simulink model "VINS"  (R2018a)
settings: Solver=FixedStepDiscrete  StartTime=0.0  StopTime=inf  FixedStep=1/Fs  RelTol=1e-3  EnableMultiTasking=on
PreLoadFcn:
  | modelDef = getModelDef(calibrateSFMA);
  | 
  | %imuPar = getImuPar('lmvpUncalibrated');
  | 
  | timeMatchThreshold = 1000;
undefined symbols (not defined in the file or in its folder): beep, dejitter_on, Fs, homogeneous3x4Transform_k_kmin1, imuLocationMm, imuPar, numStates, simData, tstamp_k_us, tstamp_kmin1_us
libraries: simulink x69, dspmtrx3 x35, dspindex x9, vrlib x7, dspstat3 x7, dspinverses x6, dspsigops x5, dspmathops x2, rtwdemowidgets x1, dspfactors x1, simulink_extras x1
(part 4 of 6)

== system VINS/measUpdate/plotVidLatency/DT convert ==
  In1 : Inport
  Data Store Read : DataStoreRead  DataStoreName=DataTypeRef
  Data Type Conversion Inherited : simulink/Signal Attributes/Data Type Conversion Inherited  ConvertRealWorld=Real World Value  DoSatur=off
      settings: SourceProductName=Simulink  SourceProductBaseCode=SL
  Out1 : Outport
  wires:
  Data Type Conversion Inherited/1 -> Out1/1
  Data Store Read/1 -> Data Type Conversion Inherited/1
  In1/1 -> Data Type Conversion Inherited/2

== system VINS/measUpdate/plotVidLatency/DT convert1 ==
  In1 : Inport
  Data Store Read : DataStoreRead  DataStoreName=DataTypeRef
  Data Type Conversion Inherited : simulink/Signal Attributes/Data Type Conversion Inherited  ConvertRealWorld=Real World Value  DoSatur=off
      settings: SourceProductName=Simulink  SourceProductBaseCode=SL
  Out1 : Outport
  wires:
  In1/1 -> Data Type Conversion Inherited/2
  Data Store Read/1 -> Data Type Conversion Inherited/1
  Data Type Conversion Inherited/1 -> Out1/1

== system VINS/measUpdate/plotVidLatency/DT convert2 ==
  In1 : Inport
  Data Store Read : DataStoreRead  DataStoreName=DataTypeRef
  Data Type Conversion Inherited : simulink/Signal Attributes/Data Type Conversion Inherited  ConvertRealWorld=Real World Value  DoSatur=off
      settings: SourceProductName=Simulink  SourceProductBaseCode=SL
  Out1 : Outport
  wires:
  In1/1 -> Data Type Conversion Inherited/2
  Data Store Read/1 -> Data Type Conversion Inherited/1
  Data Type Conversion Inherited/1 -> Out1/1

== system VINS/measUpdate/plotVidLatency/set 0x08 bit ==
  Enable : EnablePort
  Assertion : Assertion  AssertionFailFcn=disp('Unacceptable video delay >3 frames'); beep;  StopWhenAssertionFail=off
  Bit Set : simulink/Logic and Bit Operations/Bit Set  iBit=3
      settings: SourceProductName=Simulink  SourceProductBaseCode=SL
  Constant : Constant  Value=false
  Data Store Read : DataStoreRead  DataStoreName=errorBitfield
  Data Store Write : DataStoreWrite  DataStoreName=errorBitfield
  wires:
  Data Store Read/1 -> Bit Set/1
  Bit Set/1 -> Data Store Write/1
  Constant/1 -> Assertion/1

== system VINS/measUpdate/plotVidLatency/set 0x10 bit ==
  Enable : EnablePort
  Assertion : Assertion  AssertionFailFcn=disp('Unacceptable video delay >3.9 frames'); beep;  StopWhenAssertionFail=off
  Bit Set : simulink/Logic and Bit Operations/Bit Set  iBit=4
      settings: SourceProductName=Simulink  SourceProductBaseCode=SL
  Constant : Constant  Value=false
  Data Store Read : DataStoreRead  DataStoreName=errorBitfield
  Data Store Write : DataStoreWrite  DataStoreName=errorBitfield
  wires:
  Constant/1 -> Assertion/1
  Bit Set/1 -> Data Store Write/1
  Data Store Read/1 -> Bit Set/1

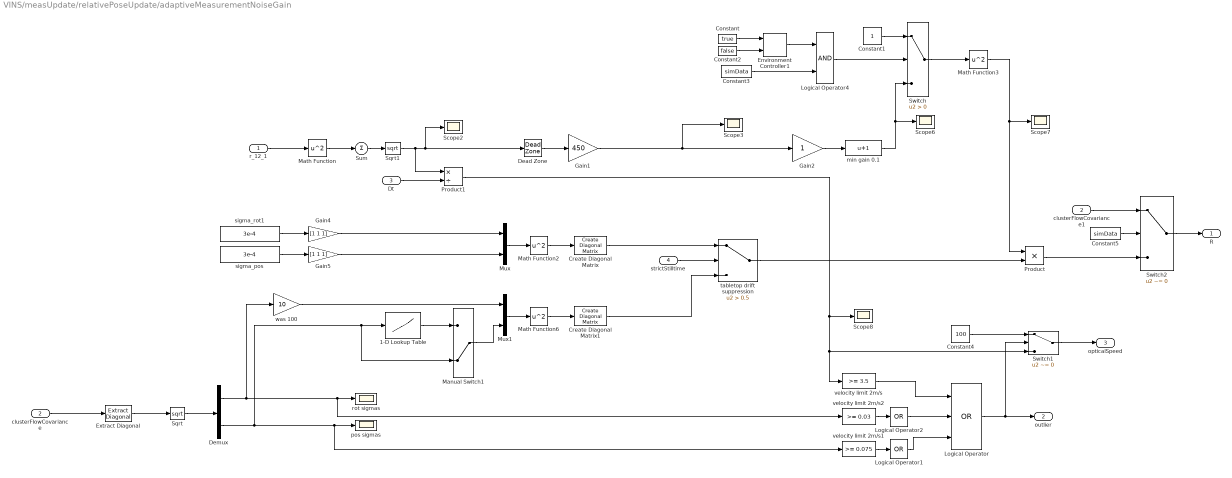
== system VINS/measUpdate/relativePoseUpdate/adaptiveMeasurementNoiseGain ==
  r_12_1 : Inport
  clusterFlowCovariance : Inport  Port=2
  Dt : Inport  Port=3
  strictStilltime : Inport  Port=4
  1-D Lookup Table : Lookup_n-D  NumberOfTableDimensions=1  BreakpointsForDimension1="[0 0.005 0.010  0.015 0.020 0.025 0.075]"  Table="[0 0.004 0.007  0.009 0.010 0.0105 0.0105]"  InternalRulePriority=Speed  RndMeth=Simplest  InputSameDT=on
  Constant : Constant  Value=true
  Constant1 : Constant
  Constant2 : Constant  Value=false
  Constant3 : Constant  Value=simData
  Constant4 : Constant  Value=100  OutDataTypeStr=Inherit: Inherit via back propagation
  Constant5 : Constant  Value=simData
  Create Diagonal Matrix : dspmtrx3/Create Diagonal Matrix
      settings: SourceProductName=DSP System Toolbox  SourceProductBaseCode=DS
  Create Diagonal Matrix1 : dspmtrx3/Create Diagonal Matrix
      settings: SourceProductName=DSP System Toolbox  SourceProductBaseCode=DS
  Dead Zone : DeadZone  LowerValue=-1e-3  UpperValue=1e-3  SaturateOnIntegerOverflow=on
  Demux : Demux  Outputs=2
  Environment Controller1 : simulink/Signal Routing/Environment Controller
      settings: SourceProductName=Simulink  SourceProductBaseCode=SL
  Extract Diagonal : dspmtrx3/Extract Diagonal
      settings: SourceProductName=DSP System Toolbox  SourceProductBaseCode=DS
  Gain1 : Gain  Gain=450
  Gain2 : Gain
  Gain4 : Gain  Gain=[1 1 1]
  Gain5 : Gain  Gain=[1 1 1]
  Logical Operator : Logic  Operator=OR  Inputs=3  AllPortsSameDT=off  OutDataTypeStr=boolean
  Logical Operator1 : Logic  Operator=OR  Inputs=1  AllPortsSameDT=off  OutDataTypeStr=boolean
  Logical Operator2 : Logic  Operator=OR  Inputs=1  AllPortsSameDT=off  OutDataTypeStr=boolean
  Logical Operator4 : Logic  AllPortsSameDT=off  OutDataTypeStr=boolean
  Manual Switch1 : ManualSwitch  CurrentSetting=0
  Math Function{,2..3,6} (4 alike) : Math  Operator=square  SaturateOnIntegerOverflow=on
  Mux : Mux  Inputs=2
  Mux1 : Mux  Inputs=2
  Product : Product
  Product1 : Product  Inputs=*/
  Scope{2..3,6..8} (5 alike) : Scope
  Sqrt : Sqrt  SaturateOnIntegerOverflow=on
  Sqrt1 : Sqrt  SaturateOnIntegerOverflow=on
  Sum : Sum  Inputs=+
  Switch : Switch  Criteria=u2 > Threshold
  Switch1 : Switch  Criteria=u2 ~= 0
  Switch2 : Switch  Criteria=u2 ~= 0
  clusterFlowCovariance1 : InportShadow  Port=2
  min gain 0.1 : Bias  Bias=1
  pos sigmas : Scope
  rot sigmas : Scope
  sigma_pos : Constant  Value=3e-4
  sigma_rot1 : Constant  Value=3e-4
  tabletop drift suppression : Switch  Criteria=u2 > Threshold  Threshold=0.5
  velocity limit 2m/s : simulink/Logic and Bit Operations/Compare To Constant  relop=>=  const=3.5  OutDataTypeStr=boolean
  velocity limit 2m/s1 : simulink/Logic and Bit Operations/Compare To Constant  relop=>=  const=0.075  OutDataTypeStr=boolean
  velocity limit 2m/s2 : simulink/Logic and Bit Operations/Compare To Constant  relop=>=  const=0.03  OutDataTypeStr=boolean
  was 100 : Gain  Gain=10
  R : Outport
  outlier : Outport  Port=2
  opticalSpeed : Outport  Port=3
  wires:
  Math Function/1 -> Sum/1
  Sum/1 -> Sqrt1/1
  Extract Diagonal/1 -> Sqrt/1
  Demux/1 -> velocity limit 2m/s2/1, rot sigmas/1, was 100/1
  r_12_1/1 -> Math Function/1
  Sqrt1/1 -> Product1/1, Dead Zone/1, Scope2/1
  Dead Zone/1 -> Gain1/1
  Switch/1 -> Math Function3/1
  Product/1 -> Switch2/3
  Math Function3/1 -> Scope7/1, Product/1
  min gain 0.1/1 -> Scope6/1, Switch/3
  Constant3/1 -> Logical Operator4/2
  Environment Controller1/1 -> Logical Operator4/1
  Constant/1 -> Environment Controller1/1
  Constant2/1 -> Environment Controller1/2
  Constant1/1 -> Switch/1
  Logical Operator4/1 -> Switch/2
  Mux/1 -> Math Function2/1
  Math Function2/1 -> Create Diagonal Matrix/1
  Gain4/1 -> Mux/1
  Gain5/1 -> Mux/2
  sigma_pos/1 -> Gain5/1
  sigma_rot1/1 -> Gain4/1
  Create Diagonal Matrix/1 -> tabletop drift suppression/1
  clusterFlowCovariance/1 -> Extract Diagonal/1
  tabletop drift suppression/1 -> Product/2
  Dt/1 -> Product1/2
  Product1/1 -> Switch1/3, velocity limit 2m/s/1, Scope8/1
  velocity limit 2m/s/1 -> Logical Operator/1
  Gain1/1 -> Gain2/1, Scope3/1
  Gain2/1 -> min gain 0.1/1
  velocity limit 2m/s2/1 -> Logical Operator2/1
  velocity limit 2m/s1/1 -> Logical Operator1/1
  Logical Operator/1 -> Switch1/2, outlier/1
  Logical Operator1/1 -> Logical Operator/3
  Logical Operator2/1 -> Logical Operator/2
  strictStilltime/1 -> tabletop drift suppression/2
  Math Function6/1 -> Create Diagonal Matrix1/1
  Mux1/1 -> Math Function6/1
  Create Diagonal Matrix1/1 -> tabletop drift suppression/3
  Sqrt/1 -> Demux/1
  was 100/1 -> Mux1/1
  Manual Switch1/1 -> Mux1/2
  1-D Lookup Table/1 -> Manual Switch1/1
  Demux/2 -> Manual Switch1/2, 1-D Lookup Table/1, velocity limit 2m/s1/1, pos sigmas/1
  Switch1/1 -> opticalSpeed/1
  Constant4/1 -> Switch1/1
  Switch2/1 -> R/1
  Constant5/1 -> Switch2/2
  clusterFlowCovariance1/1 -> Switch2/1

== system VINS/measUpdate/relativePoseUpdate/applyErrors ==
  In1 : Inport
  In2 : Inport  Port=2
  Enable : EnablePort
  Product1 : Product  Multiplication=Matrix(*)
  applyErrors : Subsystem
  wires:
  Product1/1 -> applyErrors/1(errors)  "errors"
  In1/1 -> Product1/1
  In2/1 -> Product1/2

== system VINS/measUpdate/relativePoseUpdate/formInnovation ==
  idx1 : Inport
  idx2 : Inport  Port=2
  r_c1c2_c1 : Inport  Port=3
  C_2_1 : Inport  Port=4
  C1nhat*Ccb*Cc2c1*Cbc*Cn2hat : Product  Inputs=5  Multiplication=Matrix(*)
  Data Store Read : DataStoreRead  DataStoreName=C_b_n_list
  Data Store Read1 : DataStoreRead  DataStoreName=r_b_n_list
  Data Store Read2 : DataStoreRead  DataStoreName=Ccb
  Data Store Read5 : DataStoreRead  DataStoreName=r_bc_b
  MATLAB Function1 : MATLAB Function  TreatAsAtomicUnit=on
  MATLAB Function3 : MATLAB Function  TreatAsAtomicUnit=on
  Matrix Multiply : Product  Inputs=3  Multiplication=Matrix(*)
  Matrix Multiply1 : Product  Multiplication=Matrix(*)
  Matrix Multiply2 : Product  Multiplication=Matrix(*)
  Mux : Mux  Inputs=[3 3]
  Permute Dimensions : PermuteDimensions
  Permute Dimensions1 : PermuteDimensions
  Scope{,1..3} (4 alike) : Scope
  Selector : Selector  NumberOfDimensions=3  InputPortWidth=3  IndexOptions=Select all,Select all,Index vector (port)  Indices=1:3,1:3,1  OutputSizes=1,1,1
  Selector1 : Selector  NumberOfDimensions=3  InputPortWidth=3  IndexOptions=Index vector (dialog),Index vector (dialog),Index vector (port)  Indices=1:3,1:3,1  OutputSizes=1,1,1
  Selector2 : Selector  NumberOfDimensions=3  InputPortWidth=3  IndexOptions=Index vector (dialog),Index vector (dialog),Index vector (port)  Indices=1:3,1,1  OutputSizes=1,1,1
  Selector3 : Selector  NumberOfDimensions=3  InputPortWidth=3  IndexOptions=Index vector (dialog),Index vector (dialog),Index vector (port)  Indices=1:3,1,1  OutputSizes=1,1,1
  Sum : Sum  Inputs=-+|
  Sum1 : Sum  Inputs=-++
  Sum2 : Sum  Inputs=-+|
  r_c1c2_n : Outport
  nu : Outport  Port=2
  wires:
  idx1/1 -> Selector/2, Selector2/2
  Data Store Read/1 -> Selector1/1, Selector/1
  idx2/1 -> Selector1/2, Selector3/2
  Data Store Read1/1 -> Selector3/1, Selector2/1
  Selector/1 -> C1nhat*Ccb*Cc2c1*Cbc*Cn2hat/1, Matrix Multiply2/1, Matrix Multiply/1  "C1nhat"
  C_2_1/1 -> C1nhat*Ccb*Cc2c1*Cbc*Cn2hat/3, MATLAB Function1/1(Cbn)
  Selector1/1 -> Matrix Multiply1/1, Permute Dimensions/1  "C2nhat"
  Permute Dimensions/1 -> C1nhat*Ccb*Cc2c1*Cbc*Cn2hat/5
  C1nhat*Ccb*Cc2c1*Cbc*Cn2hat/1 -> MATLAB Function3/1(Cbn)
  MATLAB Function3/1(eul) -> Mux/1, Scope/1
  Selector3/1 -> Sum/2  "r_2_n_hat"
  Selector2/1 -> Sum/1  "r_1_n_hat"
  Sum/1 -> Sum1/2  "r_b1b2_n_hat"
  r_c1c2_c1/1 -> Matrix Multiply/3, Scope3/1
  Matrix Multiply/1 -> Sum1/1, r_c1c2_n/1
  Sum1/1 -> Scope1/1, Mux/2
  Mux/1 -> nu/1
  MATLAB Function1/1(eul) -> Scope2/1
  Data Store Read2/1 -> Permute Dimensions1/1, C1nhat*Ccb*Cc2c1*Cbc*Cn2hat/2, Matrix Multiply/2
  Data Store Read5/1 -> Matrix Multiply1/2, Matrix Multiply2/2
  Matrix Multiply1/1 -> Sum2/2
  Matrix Multiply2/1 -> Sum2/1
  Sum2/1 -> Sum1/3
  Permute Dimensions1/1 -> C1nhat*Ccb*Cc2c1*Cbc*Cn2hat/4

== system VINS/measUpdate/relativePoseUpdate/formMeasurementMatrix ==
  rows1 : Inport
  rows2 : Inport  Port=2
  r_c1c2_n : Inport  Port=3
  Assignment : Assignment  NumberOfDimensions=2  DiagnosticForDimensions=Warning  IndexOptions=Assign all,Index vector (port)  Indices=1,1  OutputSizes=1,1
  Assignment1 : Assignment  NumberOfDimensions=2  DiagnosticForDimensions=Warning  IndexOptions=Assign all,Index vector (port)  Indices=1,1  OutputSizes=1,1
  Assignment2 : Assignment  NumberOfDimensions=2  DiagnosticForDimensions=Warning  IndexOptions=Index vector (dialog),Index vector (dialog)  Indices=4:6,1:3  OutputSizes=1,1
  Assignment3 : Assignment  NumberOfDimensions=2  DiagnosticForDimensions=Warning  IndexOptions=Index vector (dialog),Index vector (dialog)  Indices=4:6,1:3  OutputSizes=1,1
  Constant : Constant  Value=-eye(6)  OutDataTypeStr=Inherit: Inherit via back propagation
  Constant1 : Constant  Value=zeros(6, 6*modelDef.maxNumDelayedPoses)  OutDataTypeStr=Inherit: Inherit via back propagation
  Constant2 : Constant  Value=eye(6)  OutDataTypeStr=Inherit: Inherit via back propagation
  Data Store Read : DataStoreRead  DataStoreName=r_bc_b
  Gain : Gain  Gain=-1
  Hx : Constant  Value=zeros(6, modelDef.numStates)  VectorParams1D=off  OutDataTypeStr=Inherit: Inherit via back propagation
  Matrix Concatenate : Concatenate  Mode=Multidimensional array  ConcatenateDimension=2
  Sum : Sum  Inputs=|++
  skew : MATLAB Function  TreatAsAtomicUnit=on
  skew1 : MATLAB Function  TreatAsAtomicUnit=on
  Out1 : Outport
  wires:
  Matrix Concatenate/1 -> Out1/1
  Hx/1 -> Matrix Concatenate/1
  Assignment1/1 -> Matrix Concatenate/2
  Constant1/1 -> Assignment/1
  rows1/1 -> Assignment/3
  Assignment/1 -> Assignment1/1
  rows2/1 -> Assignment1/3
  Constant/1 -> Assignment2/1
  Assignment3/1 -> Assignment1/2
  skew/1(res) -> Sum/1
  Assignment2/1 -> Assignment/2
  r_c1c2_n/1 -> skew/1(inp_vr)
  Constant2/1 -> Assignment3/1
  Data Store Read/1 -> skew1/1(inp_vr)
  skew1/1(res) -> Sum/2, Assignment3/2
  Gain/1 -> Assignment2/2
  Sum/1 -> Gain/1

== system VINS/measUpdate/relativePoseUpdate/get row indices ==
  idx1 : Inport
  idx2 : Inport  Port=2
  Bias2 : Bias  Bias=(1:6)
  Bias4 : Bias  Bias=(1:6)
  Constant2 : Constant  Value=uint8(1)
  Constant3 : Constant  Value=uint8(1)
  Gain : Gain  Gain=6  OutDataTypeStr=Inherit: Same as input
  Gain1 : Gain  Gain=6  OutDataTypeStr=Inherit: Same as input
  Scope4 : Scope
  Scope5 : Scope
  Sum1 : Sum  Inputs=|+-
  Sum2 : Sum  Inputs=|+-
  validateRecency : Subsystem  Commented=on
  rows1 : Outport
  rows2 : Outport  Port=2
  valid : Outport  Port=3
  wires:
  idx2/1 -> Scope5/1, validateRecency/2(In2), Sum2/1
  idx1/1 -> Scope4/1, validateRecency/1(In1), Sum1/1
  Gain/1 -> Bias2/1
  Bias2/1 -> rows1/1
  Gain1/1 -> Bias4/1
  Bias4/1 -> rows2/1
  Constant2/1 -> Sum1/2
  Sum1/1 -> Gain/1
  Sum2/1 -> Gain1/1
  Constant3/1 -> Sum2/2
  validateRecency/1(valid) -> valid/1

== system VINS/measUpdate/relativePoseUpdate/updateCovariance ==
  note: This repairs the covariance matrix by adding the smallest E matrix to it to make it positive definite.
  K : Inport
  P : Inport  Port=2
  H : Inport  Port=3
  R : Inport  Port=4
  Enable : EnablePort
  Data Store Write : DataStoreWrite  DataStoreName=Pxx
  Data Store Write1 : DataStoreWrite  DataStoreName=Pxc
  Data Store Write2 : DataStoreWrite  DataStoreName=Pcc
  Matrix 1-Norm1 : dspmtrx3/Matrix  1-Norm  roundingMode=Floor  overflowMode=off  outputDataTypeStr=Inherit: Same as accumulator  outputMin=[]  outputMax=[]  outputLastDataTypeStr=Inherit: Same as accumulator
      settings: SourceProductName=DSP System Toolbox  SourceProductBaseCode=DS
  Matrix Multiply : Product  Inputs=3  Multiplication=Matrix(*)
  Permute Dimensions : PermuteDimensions
  Scope1 : Scope
  Submatrix3 : dspmtrx3/Submatrix  RowSpan=Range of rows  RowStartMode=First  RowStartIndex=1  RowEndMode=Index  RowEndIndex=modelDef.numStates  ColSpan=Range of columns  ColStartMode=First  ColStartIndex=1  ColEndMode=Index  ColEndIndex=modelDef.numStates
  Submatrix4 : dspmtrx3/Submatrix  RowSpan=Range of rows  RowStartMode=First  RowStartIndex=1  RowEndMode=Index  RowEndIndex=modelDef.numStates  ColSpan=Range of columns  ColStartMode=Index  ColStartIndex=modelDef.numStates + 1  ColEndMode=Last  ColEndIndex=1
  Submatrix5 : dspmtrx3/Submatrix  RowSpan=Range of rows  RowStartMode=Index  RowStartIndex=modelDef.numStates + 1  RowEndMode=Last  RowEndIndex=modelDef.numStates  ColSpan=Range of columns  ColStartMode=Index  ColStartIndex=modelDef.numStates + 1  ColEndMode=Last  ColEndIndex=1
  josephCovarianceUpdate : MATLAB Function  TreatAsAtomicUnit=on
  modifiedCholesky : MATLAB Function  TreatAsAtomicUnit=on
  repairCovarianceAndWrite : Subsystem  Commented=on  TreatAsAtomicUnit=on
      settings: RTWSystemCode=Nonreusable function  RTWFcnNameOpts=Use subsystem name
  writeCovariances : Subsystem  Commented=on  TreatAsAtomicUnit=on
  wires:
  P/1 -> josephCovarianceUpdate/1(P)
  R/1 -> josephCovarianceUpdate/4(R)
  H/1 -> josephCovarianceUpdate/3(H)
  K/1 -> josephCovarianceUpdate/2(K)
  Permute Dimensions/1 -> Matrix Multiply/3
  josephCovarianceUpdate/1(Pplus) -> modifiedCholesky/1(G), repairCovarianceAndWrite/1(In1), writeCovariances/1(In1)
  modifiedCholesky/1(L) -> Permute Dimensions/1, Matrix Multiply/1
  modifiedCholesky/2(D) -> Matrix Multiply/2
  modifiedCholesky/3(E) -> Matrix 1-Norm1/1
  Matrix 1-Norm1/1 -> Scope1/1
  Submatrix5/1 -> Data Store Write2/1
  Submatrix4/1 -> Data Store Write1/1
  Submatrix3/1 -> Data Store Write/1
  Matrix Multiply/1 -> Submatrix5/1, Submatrix4/1, Submatrix3/1

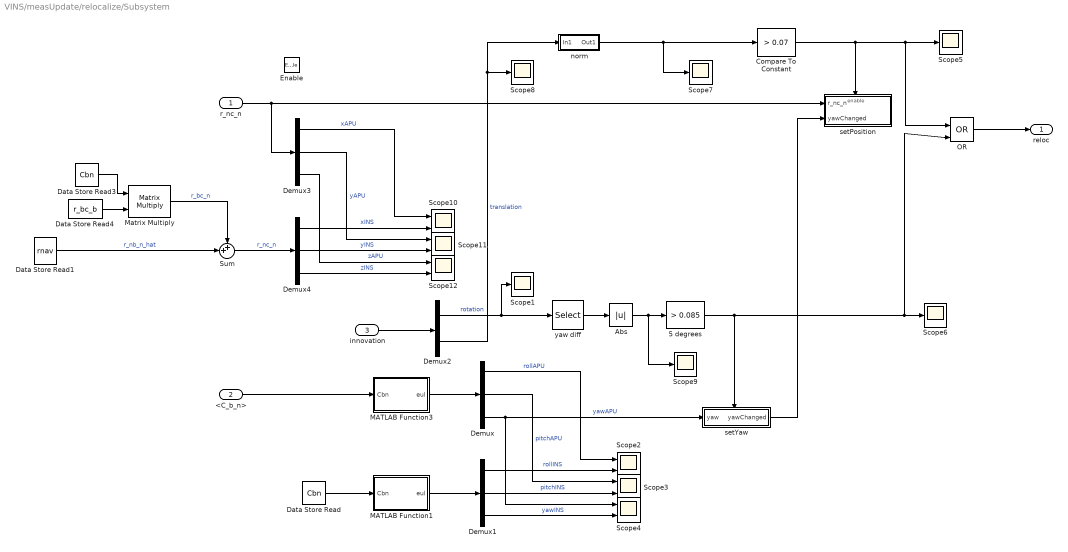
== system VINS/measUpdate/relocalize/Subsystem ==
  r_nc_n : Inport
  <C_b_n> : Inport  Port=2
  innovation : Inport  Port=3
  Enable : EnablePort
  5 degrees : simulink/Logic and Bit Operations/Compare To Constant  relop=>  const=0.085  OutDataTypeStr=boolean
  Abs : Abs
  Compare To Constant : simulink/Logic and Bit Operations/Compare To Constant  relop=>  const=0.07  OutDataTypeStr=boolean
  Data Store Read : DataStoreRead  DataStoreName=Cbn
  Data Store Read1 : DataStoreRead  DataStoreName=rnav
  Data Store Read3 : DataStoreRead  DataStoreName=Cbn
  Data Store Read4 : DataStoreRead  DataStoreName=r_bc_b
  Demux{,1,3..4} (4 alike) : Demux  Outputs=3
  Demux2 : Demux  Outputs=[3 3]
  MATLAB Function1 : MATLAB Function  TreatAsAtomicUnit=on
  MATLAB Function3 : MATLAB Function  TreatAsAtomicUnit=on
  Matrix Multiply : Product  Multiplication=Matrix(*)
  OR : Logic  Operator=OR  IconShape=distinctive  AllPortsSameDT=off  OutDataTypeStr=boolean
  Scope{1,5..9} (6 alike) : Scope
  Scope{2..4,10..12} (6 alike) : Scope  NumInputPorts=2
  Sum : Sum  Inputs=++|
  norm : Subsystem  TreatAsAtomicUnit=on
  setPosition : Subsystem  TreatAsAtomicUnit=on
  setYaw : Subsystem  TreatAsAtomicUnit=on
  yaw diff : Selector  InputPortWidth=3  IndexOptions=Index vector (dialog)  Indices=3  OutputSizes=1
  reloc : Outport  OutputWhenDisabled=reset  InitialOutput=false
  wires:
  norm/1(Out1) -> Scope7/1, Compare To Constant/1
  yaw diff/1 -> Abs/1
  Demux1/1 -> Scope2/2  "rollINS"
  Demux1/2 -> Scope3/2  "pitchINS"
  5 degrees/1 -> Scope6/1, OR/2, setYaw/Enable
  Data Store Read/1 -> MATLAB Function1/1(Cbn)
  MATLAB Function1/1(eul) -> Demux1/1
  Demux/3 -> Scope4/1, setYaw/1(yaw)  "yawAPU"
  Demux2/2 -> Scope8/1, norm/1(In1)  "translation"
  Demux/2 -> Scope3/1  "pitchAPU"
  Demux2/1 -> yaw diff/1, Scope1/1  "rotation"
  Demux1/3 -> Scope4/2  "yawINS"
  OR/1 -> reloc/1
  Demux/1 -> Scope2/1  "rollAPU"
  MATLAB Function3/1(eul) -> Demux/1
  innovation/1 -> Demux2/1
  <C_b_n>/1 -> MATLAB Function3/1(Cbn)
  Compare To Constant/1 -> setPosition/Enable, OR/1, Scope5/1
  Demux3/3 -> Scope12/1  "zAPU"
  Demux3/1 -> Scope10/1  "xAPU"
  Sum/1 -> Demux4/1  "r_nc_n"
  Demux4/3 -> Scope12/2  "zINS"
  Demux4/1 -> Scope10/2  "xINS"
  Demux4/2 -> Scope11/2  "yINS"
  Demux3/2 -> Scope11/1  "yAPU"
  r_nc_n/1 -> Demux3/1, setPosition/1(r_nc_n)
  Abs/1 -> Scope9/1, 5 degrees/1
  Data Store Read1/1 -> Sum/2  "r_nb_n_hat"
  Data Store Read3/1 -> Matrix Multiply/1
  Data Store Read4/1 -> Matrix Multiply/2
  Matrix Multiply/1 -> Sum/1  "r_bc_n"
  setYaw/1(yawChanged) -> setPosition/2(yawChanged)

== system VINS/measUpdate/wipe out delayed states/setP ==
  Enable : EnablePort
  Constant : Constant  Value=zeros(modelDef.numStates, modelDef.statesPerDelayedPose*modelDef.maxNumDelayedPoses)  OutDataTypeStr=Inherit: Inherit via back propagation
  Constant1 : Constant  Value=zeros(modelDef.statesPerDelayedPose*modelDef.maxNumDelayedPoses, modelDef.statesPerDelayedPose*modelDef.maxNumDelayedPoses)  OutDataTypeStr=Inherit: Inherit via back propagation
  DT police1 : Subsystem  TreatAsAtomicUnit=on
  DT police2 : Subsystem  TreatAsAtomicUnit=on
  DT police3 : Subsystem  TreatAsAtomicUnit=on
  Data Store Read : DataStoreRead  DataStoreName=Pxx
  Data Store Write : DataStoreWrite  DataStoreName=Pxx
  Data Store Write1 : DataStoreWrite  DataStoreName=Pxc
  Data Store Write2 : DataStoreWrite  DataStoreName=Pcc
  MATLAB Function1 : MATLAB Function  TreatAsAtomicUnit=on
  Submatrix : dspmtrx3/Submatrix  RowSpan=Range of rows  RowStartMode=Index  RowStartIndex=4  RowEndMode=Index  RowEndIndex=6  ColSpan=Range of columns  ColStartMode=Index  ColStartIndex=4  ColEndMode=Index  ColEndIndex=6
  Submatrix1 : dspmtrx3/Submatrix  RowSpan=Range of rows  RowStartMode=Index  RowStartIndex=13  RowEndMode=Index  RowEndIndex=15  ColSpan=Range of columns  ColStartMode=Index  ColStartIndex=13  ColEndMode=Index  ColEndIndex=15
  "initial position error, m rms" : Constant  Value=[0.01; 0.01; 0.01]  VectorParams1D=off  OutDataTypeStr=Inherit: Inherit via back propagation
  "initial rotation error, rad rms" : Constant  Value=[0.1; 0.1; 0.1]  VectorParams1D=off  OutDataTypeStr=Inherit: Inherit via back propagation
  "initial vel error, m/s" : Constant  Value=[1; 1; 1]  VectorParams1D=off  OutDataTypeStr=Inherit: Inherit via back propagation
  wires:
  "initial position error, m rms"/1 -> DT police2/1(In1), MATLAB Function1/2(initialPosUncert)
  "initial rotation error, rad rms"/1 -> DT police1/1(In1), MATLAB Function1/1(initialRotUncert)
  MATLAB Function1/1(P0) -> Data Store Write/1
  Constant/1 -> Data Store Write1/1
  Constant1/1 -> Data Store Write2/1
  "initial vel error, m/s"/1 -> DT police3/1(In1), MATLAB Function1/3(initialVelUncert)
  Data Store Read/1 -> Submatrix1/1, Submatrix/1
  Submatrix/1 -> MATLAB Function1/4(gyroBiasCov)  "gyroBiasCov"
  Submatrix1/1 -> MATLAB Function1/5(accelBiasCov)

== system VINS/measUpdate/zuptMeasUpdate/DT police ==
  In1 : Inport
  Data Store Read : DataStoreRead  DataStoreName=DataTypeRef
  Data Type Duplicate : DataTypeDuplicate
  wires:
  Data Store Read/1 -> Data Type Duplicate/1
  In1/1 -> Data Type Duplicate/2

== system VINS/measUpdate/zuptMeasUpdate/DT police1 ==
  In1 : Inport
  Data Store Read : DataStoreRead  DataStoreName=DataTypeRef
  Data Type Duplicate : DataTypeDuplicate
  wires:
  In1/1 -> Data Type Duplicate/2
  Data Store Read/1 -> Data Type Duplicate/1

== system VINS/measUpdate/zuptMeasUpdate/applyErrors ==
  errorStateEstimates : Inport
  Constant : Constant  Value=modelDef.trackGyroSfma
  Constant1 : Constant  Value=modelDef.trackAccelSfma
  Constant2 : Constant  Value=modelDef.trackAccelBiases
  Constant3 : Constant  Value=modelDef.trackGyroGsens
  Data Store Read1 : DataStoreRead  DataStoreName=dw
  Data Store Read2 : DataStoreRead  DataStoreName=Cbn
  Data Store Read3 : DataStoreRead  DataStoreName=rnav
  Data Store Read4 : DataStoreRead  DataStoreName=vnav
  Data Store Write1 : DataStoreWrite  DataStoreName=Cbn
  Data Store Write2 : DataStoreWrite  DataStoreName=dw
  Data Store Write3 : DataStoreWrite  DataStoreName=rnav
  Data Store Write4 : DataStoreWrite  DataStoreName=vnav
  Multiport Selector : dspindex/Multiport Selector  rowsOrCols=Rows  idxCellArray={ 1:3, 4:6, 7:9, 10:12, 13:15, 16:24, 25:33, 34:42 }  idxErrMode=Clip Index
  Product2 : Product  Multiplication=Matrix(*)
  Scope{,1..3} (4 alike) : Scope
  Sum : Sum  Inputs=++|
  Sum1 : Sum  Inputs=++|
  Sum2 : Sum  Inputs=-+|
  Sum3 : Sum  Inputs=-+|
  reOrthonormalization : Subsystem  TreatAsAtomicUnit=on
  skew : MATLAB Function  TreatAsAtomicUnit=on
  updateAccelBiases : Subsystem
  updateAccelSfma : Subsystem
  updateGyroGsensitivity : Subsystem
  updateGyroSfma : Subsystem
  wires:
  Multiport Selector/8 -> updateGyroGsensitivity/1(In1)
  Constant3/1 -> updateGyroGsensitivity/Enable
  Constant2/1 -> updateAccelBiases/Enable
  Multiport Selector/5 -> Scope3/1, updateAccelBiases/1(In1)
  Multiport Selector/7 -> updateAccelSfma/1(In1)
  Constant1/1 -> updateAccelSfma/Enable
  Multiport Selector/6 -> updateGyroSfma/1(In1)
  Constant/1 -> updateGyroSfma/Enable
  skew/1(res) -> Product2/1  "[phi X]"
  Product2/1 -> Sum/1
  Sum/1 -> reOrthonormalization/1(In1)
  Data Store Read2/1 -> Product2/2, Sum/2
  reOrthonormalization/1(Out1) -> Data Store Write1/1
  Multiport Selector/1 -> skew/1(inp_vr)  "phi rotation errors"
  Data Store Read1/1 -> Sum1/2
  Sum1/1 -> Data Store Write2/1
  Multiport Selector/2 -> Scope/1, Sum1/1  "gyro bias errors"
  errorStateEstimates/1 -> Multiport Selector/1
  Sum2/1 -> Data Store Write3/1
  Data Store Read3/1 -> Sum2/2
  Data Store Read4/1 -> Sum3/2
  Sum3/1 -> Data Store Write4/1
  Multiport Selector/3 -> Scope1/1, Sum2/1
  Multiport Selector/4 -> Scope2/1, Sum3/1

== system VINS/reportOutputs/updateDistTravelled/increment distTravelled ==
  deltaPos : Inport
  Enable : EnablePort
  Data Store Read : DataStoreRead  DataStoreName=distTravelled
  Data Store Write : DataStoreWrite  DataStoreName=distTravelled
  Sum : Sum  Inputs=|++
  distTravelled : Outport  InitialOutput=0
  wires:
  Data Store Read/1 -> Sum/1
  Sum/1 -> distTravelled/1, Data Store Write/1
  deltaPos/1 -> Sum/2

== system VINS/reportOutputs/updateDistTravelled/latch ==
  In1 : Inport
  Enable : EnablePort
  Out1 : Outport  InitialOutput=0
  wires:
  In1/1 -> Out1/1

== system VINS/sensorCompensation/detectAccelSaturation/set 0x01 bit ==
  Enable : EnablePort
  Assertion : Assertion  AssertionFailFcn=disp('accel_clip'); beep;  StopWhenAssertionFail=off
  Bit Set : simulink/Logic and Bit Operations/Bit Set  iBit=0
      settings: SourceProductName=Simulink  SourceProductBaseCode=SL
  Constant : Constant  Value=false
  Data Store Read : DataStoreRead  DataStoreName=errorBitfield
  Data Store Write : DataStoreWrite  DataStoreName=errorBitfield
  wires:
  Constant/1 -> Assertion/1
  Bit Set/1 -> Data Store Write/1
  Data Store Read/1 -> Bit Set/1

== system VINS/sensorCompensation/detectGyroSaturation/set 0x02 bit ==
  Enable : EnablePort
  Assertion : Assertion
  Bit Set : simulink/Logic and Bit Operations/Bit Set  iBit=1
      settings: SourceProductName=Simulink  SourceProductBaseCode=SL
  Constant : Constant  Value=false
  Data Store Read : DataStoreRead  DataStoreName=errorBitfield
  Data Store Write : DataStoreWrite  DataStoreName=errorBitfield
  wires:
  Data Store Read/1 -> Bit Set/1
  Bit Set/1 -> Data Store Write/1
  Constant/1 -> Assertion/1

== system VINS/uncomment and set zero noise for verification/update pure optical pose/DT police ==
  In1 : Inport
  Data Store Read : DataStoreRead  DataStoreName=DataTypeRef
  Data Type Duplicate : DataTypeDuplicate
  wires:
  Data Store Read/1 -> Data Type Duplicate/1
  In1/1 -> Data Type Duplicate/2

== system VINS/uncomment and set zero noise for verification/update pure optical pose/initialize H ==
  Enable : EnablePort
  Constant : Constant  Value=[0 0 0 1]  VectorParams1D=off  OutDataTypeStr=Inherit: Inherit via back propagation
  Constant9 : Constant  Value=imuLocationMm  OutDataTypeStr=Inherit: Inherit via back propagation
  Data Store Read : DataStoreRead  DataStoreName=Cbn
  Data Store Read1 : DataStoreRead  DataStoreName=rnav
  Data Store Write : DataStoreWrite  DataStoreName=H
  Gain : Gain  Gain=1/1000
  Matrix Concatenate : Concatenate  Mode=Multidimensional array  ConcatenateDimension=2
  Matrix Concatenate1 : Concatenate  Mode=Multidimensional array
  Matrix Multiply : Product  Multiplication=Matrix(*)
  Sum : Sum  Inputs=-+|
  wires:
  Constant/1 -> Matrix Concatenate1/2
  Sum/1 -> Matrix Concatenate/2  "r_nc_n"
  Matrix Concatenate/1 -> Matrix Concatenate1/1
  Matrix Concatenate1/1 -> Data Store Write/1
  Data Store Read1/1 -> Sum/2  "r_nb_n"
  Constant9/1 -> Gain/1
  Matrix Multiply/1 -> Sum/1  "r_cb_n"
  Data Store Read/1 -> Matrix Multiply/1, Matrix Concatenate/1  "Ccn = Cbn"
  Gain/1 -> Matrix Multiply/2  "r_cb_c"

== system VINS/initStatesCovariances/realInit/calcCbn/DT convert ==
  In1 : Inport
  Data Store Read : DataStoreRead  DataStoreName=DataTypeRef
  Data Type Conversion Inherited : simulink/Signal Attributes/Data Type Conversion Inherited  ConvertRealWorld=Real World Value  DoSatur=off
      settings: SourceProductName=Simulink  SourceProductBaseCode=SL
  Out1 : Outport
  wires:
  Data Type Conversion Inherited/1 -> Out1/1
  Data Store Read/1 -> Data Type Conversion Inherited/1
  In1/1 -> Data Type Conversion Inherited/2

== system VINS/initStatesCovariances/realInit/calcCbn/DT convert1 ==
  In1 : Inport
  Data Store Read : DataStoreRead  DataStoreName=DataTypeRef
  Data Type Conversion Inherited : simulink/Signal Attributes/Data Type Conversion Inherited  ConvertRealWorld=Real World Value  DoSatur=off
      settings: SourceProductName=Simulink  SourceProductBaseCode=SL
  Out1 : Outport
  wires:
  In1/1 -> Data Type Conversion Inherited/2
  Data Store Read/1 -> Data Type Conversion Inherited/1
  Data Type Conversion Inherited/1 -> Out1/1

== system VINS/initStatesCovariances/realInit/calcCbn/DT police ==
  In1 : Inport
  Data Store Read : DataStoreRead  DataStoreName=DataTypeRef
  Data Type Duplicate : DataTypeDuplicate
  wires:
  Data Store Read/1 -> Data Type Duplicate/1
  In1/1 -> Data Type Duplicate/2

== system VINS/initStatesCovariances/realInit/calcCbn/DT police2 ==
  In1 : Inport
  Data Store Read : DataStoreRead  DataStoreName=DataTypeRef
  Data Type Duplicate : DataTypeDuplicate
  wires:
  Data Store Read/1 -> Data Type Duplicate/1
  In1/1 -> Data Type Duplicate/2

== system VINS/initStatesCovariances/realInit/setStates/DT police ==
  In1 : Inport
  Data Store Read : DataStoreRead  DataStoreName=DataTypeRef
  Data Type Duplicate : DataTypeDuplicate
  wires:
  Data Store Read/1 -> Data Type Duplicate/1
  In1/1 -> Data Type Duplicate/2

== system VINS/initStatesCovariances/realInit/setStates/DT police1 ==
  In1 : Inport
  Data Store Read : DataStoreRead  DataStoreName=DataTypeRef
  Data Type Duplicate : DataTypeDuplicate
  wires:
  In1/1 -> Data Type Duplicate/2
  Data Store Read/1 -> Data Type Duplicate/1

== system VINS/initStatesCovariances/realInit/setStates/DT police2 ==
  In1 : Inport
  Data Store Read : DataStoreRead  DataStoreName=DataTypeRef
  Data Type Duplicate : DataTypeDuplicate
  wires:
  Data Store Read/1 -> Data Type Duplicate/1
  In1/1 -> Data Type Duplicate/2

== system VINS/initStatesCovariances/realInit/setStates/DT police3 ==
  In1 : Inport
  Data Store Read : DataStoreRead  DataStoreName=DataTypeRef
  Data Type Duplicate : DataTypeDuplicate
  wires:
  Data Store Read/1 -> Data Type Duplicate/1
  In1/1 -> Data Type Duplicate/2

== system VINS/initStatesCovariances/realInit/setStates/reOrthonormalization ==
  note: Cfixed = C + 0.5(I-CC')C
  note: from http://www.dtic.mil/dtic/tr/fulltext/u2/p003621.pdf page 12
  In1 : Inport
  C*C' : Product  Multiplication=Matrix(*)
  C*C'1 : Product  Multiplication=Matrix(*)
  Constant : Constant  Value=eye(3)  OutDataTypeStr=Inherit: Inherit via back propagation
  Gain : Gain  Gain=1/2
  Permute Dimensions : PermuteDimensions
  Sum : Sum  Inputs=|++
  Sum1 : Sum  Inputs=|+-
  Out1 : Outport
  wires:
  C*C'1/1 -> Gain/1
  Sum1/1 -> C*C'1/1
  Gain/1 -> Sum/2
  Constant/1 -> Sum1/1
  C*C'/1 -> Sum1/2
  Permute Dimensions/1 -> C*C'/2
  Sum/1 -> Out1/1
  In1/1 -> Sum/1, C*C'1/2, C*C'/1, Permute Dimensions/1

== system VINS/measUpdate/absolutePoseUpdate/applyErrors/For Each Subsystem ==
  delayedPoseCorrections : Inport  Partition=on  PartitionDimension=1  PartitionWidth=6  PartitionOffset=0
  C_c_n_list_in : Inport  Port=2  Partition=on  PartitionDimension=3  PartitionWidth=1  PartitionOffset=0
  r_c_n_list_in : Inport  Port=3  Partition=on  PartitionDimension=3  PartitionWidth=1  PartitionOffset=0
  Demux : Demux  Outputs=[3 3]
  For Each : ForEach  DisableCoverage=on  IndexMode=One-based
  Product2 : Product  Multiplication=Matrix(*)
  Sum : Sum  Inputs=++|
  Sum2 : Sum  Inputs=-+|
  reOrthonormalization : Subsystem  TreatAsAtomicUnit=on
  skew : MATLAB Function  TreatAsAtomicUnit=on
  C_c_n_list : Outport  ConcatenationDimension=3
  r_c_n_list : Outport  Port=2  ConcatenationDimension=3
  wires:
  Sum/1 -> reOrthonormalization/1(In1)
  Demux/2 -> Sum2/1
  Demux/1 -> skew/1(inp_vr)  "phi rotation errors"
  r_c_n_list_in/1 -> Sum2/2
  Sum2/1 -> r_c_n_list/1
  skew/1(res) -> Product2/1  "[phi X]"
  reOrthonormalization/1(Out1) -> C_c_n_list/1
  C_c_n_list_in/1 -> Product2/2, Sum/2
  Product2/1 -> Sum/1
  delayedPoseCorrections/1 -> Demux/1

== system VINS/measUpdate/absolutePoseUpdate/applyErrors/applyXstateErrors ==
  errorStateEstimates : Inport
  Constant : Constant  Value=modelDef.trackGyroSfma
  Constant1 : Constant  Value=modelDef.trackAccelSfma
  Constant2 : Constant  Value=modelDef.trackAccelBiases
  Constant3 : Constant  Value=modelDef.trackGyroGsens
  Data Store Read1 : DataStoreRead  DataStoreName=dw
  Data Store Read2 : DataStoreRead  DataStoreName=Cbn
  Data Store Read3 : DataStoreRead  DataStoreName=rnav
  Data Store Read4 : DataStoreRead  DataStoreName=vnav
  Data Store Write1 : DataStoreWrite  DataStoreName=Cbn
  Data Store Write2 : DataStoreWrite  DataStoreName=dw
  Data Store Write3 : DataStoreWrite  DataStoreName=rnav
  Data Store Write4 : DataStoreWrite  DataStoreName=vnav
  Multiport Selector : dspindex/Multiport Selector  rowsOrCols=Rows  idxCellArray={ 1:3, 4:6, 7:9, 10:12, 13:15, 16:24, 25:33, 34:42 }  idxErrMode=Clip Index
  Product2 : Product  Multiplication=Matrix(*)
  Scope{,1..3} (4 alike) : Scope
  Sum : Sum  Inputs=++|
  Sum1 : Sum  Inputs=++|
  Sum2 : Sum  Inputs=-+|
  Sum3 : Sum  Inputs=-+|
  reOrthonormalization : Subsystem  TreatAsAtomicUnit=on
  skew : MATLAB Function  TreatAsAtomicUnit=on
  updateAccelBiases : Subsystem
  updateAccelSfma : Subsystem
  updateGyroGsensitivity : Subsystem
  updateGyroSfma : Subsystem
  wires:
  Multiport Selector/8 -> updateGyroGsensitivity/1(In1)
  Constant3/1 -> updateGyroGsensitivity/Enable
  Constant2/1 -> updateAccelBiases/Enable
  Multiport Selector/5 -> Scope3/1, updateAccelBiases/1(In1)
  Multiport Selector/7 -> updateAccelSfma/1(In1)
  Constant1/1 -> updateAccelSfma/Enable
  Multiport Selector/6 -> updateGyroSfma/1(In1)
  Constant/1 -> updateGyroSfma/Enable
  skew/1(res) -> Product2/1  "[phi X]"
  Product2/1 -> Sum/1
  Sum/1 -> reOrthonormalization/1(In1)
  Data Store Read2/1 -> Product2/2, Sum/2
  reOrthonormalization/1(Out1) -> Data Store Write1/1
  Multiport Selector/1 -> skew/1(inp_vr)  "phi rotation errors"
  Data Store Read1/1 -> Sum1/2
  Sum1/1 -> Data Store Write2/1
  Multiport Selector/2 -> Scope/1, Sum1/1  "gyro bias errors"
  errorStateEstimates/1 -> Multiport Selector/1
  Sum2/1 -> Data Store Write3/1
  Data Store Read3/1 -> Sum2/2
  Data Store Read4/1 -> Sum3/2
  Sum3/1 -> Data Store Write4/1
  Multiport Selector/3 -> Scope1/1, Sum2/1
  Multiport Selector/4 -> Scope2/1, Sum3/1

== system VINS/measUpdate/commanded reloc/setPosition1/DT police3 ==
  In1 : Inport
  Data Store Read : DataStoreRead  DataStoreName=DataTypeRef
  Data Type Duplicate : DataTypeDuplicate
  wires:
  Data Store Read/1 -> Data Type Duplicate/1
  In1/1 -> Data Type Duplicate/2

== system VINS/measUpdate/compass meas update/update the Cbn with the errors/re-orthonormalization ==
  note: from http://www.dtic.mil/dtic/tr/fulltext/u2/p003621.pdf page 12
  note: Cfixed = C + 0.5(I-CC')C
  In1 : Inport
  C*C' : Product  Multiplication=Matrix(*)
  C*C'1 : Product  Multiplication=Matrix(*)
  Constant : Constant  Value=eye(3)
  Display : Display
  Gain : Gain  Gain=1/2
  Permute Dimensions : PermuteDimensions
  Sum : Sum  Inputs=|++
  Sum1 : Sum  Inputs=|+-
  Out1 : Outport
  wires:
  In1/1 -> Permute Dimensions/1, C*C'/1, C*C'1/2, Sum/1
  Sum/1 -> Display/1, Out1/1
  Permute Dimensions/1 -> C*C'/2
  C*C'/1 -> Sum1/2
  Constant/1 -> Sum1/1
  Gain/1 -> Sum/2
  Sum1/1 -> C*C'1/1
  C*C'1/1 -> Gain/1

== system VINS/measUpdate/gravity meas update/update the Cbn and b_g with the errors/re-orthonormalization ==
  note: Cfixed = C + 0.5(I-CC')C
  note: from http://www.dtic.mil/dtic/tr/fulltext/u2/p003621.pdf page 12
  In1 : Inport
  C*C' : Product  Multiplication=Matrix(*)
  C*C'1 : Product  Multiplication=Matrix(*)
  Constant : Constant  Value=eye(3)
  Gain : Gain  Gain=1/2
  Permute Dimensions : PermuteDimensions
  Sum : Sum  Inputs=|++
  Sum1 : Sum  Inputs=|+-
  Out1 : Outport
  wires:
  C*C'1/1 -> Gain/1
  Sum1/1 -> C*C'1/1
  Gain/1 -> Sum/2
  Constant/1 -> Sum1/1
  C*C'/1 -> Sum1/2
  Permute Dimensions/1 -> C*C'/2
  Sum/1 -> Out1/1
  In1/1 -> Sum/1, C*C'1/2, C*C'/1, Permute Dimensions/1

== system VINS/measUpdate/relativePoseUpdate/applyErrors/applyErrors ==
  errors : Inport
  Data Store Read : DataStoreRead  DataStoreName=C_b_n_list
  Data Store Read1 : DataStoreRead  DataStoreName=r_b_n_list
  Data Store Write : DataStoreWrite  DataStoreName=C_b_n_list
  Data Store Write1 : DataStoreWrite  DataStoreName=r_b_n_list
  For Each Subsystem : Subsystem  TreatAsAtomicUnit=on
  Pad : dspsigops/Pad  padAlong=Columns  dimsToPad=1  valSrc=Specify via dialog  padVal=0  spec=Output size  padNumOutRowsSpecMethod=User-specified  numOutRows=max(12, 6*modelDef.maxNumDelayedPoses)  padNumOutColsSpecMethod=User-specified  numOutCols=1  isVarDimsMode=off  padBeginning=0  padEnd=0  outSizeMode=User-specified  outSize=1  padSigAt=End  trunc_flag=None  roundingMode=Floor  overflowMode=off  truncOrWrapMode=Truncate  wrap_flag=None
      settings: SourceProductName=DSP System Toolbox  SourceProductBaseCode=DS
  Selector : Selector  NumberOfDimensions=2  InputPortWidth=3  IndexOptions=Starting index (dialog),Index vector (dialog)  Indices=1,1  OutputSizes=modelDef.numStates,modelDef.numStates
  Selector1 : Selector  NumberOfDimensions=2  InputPortWidth=3  IndexOptions=Starting index (dialog),Index vector (dialog)  Indices=modelDef.numStates+1,1  OutputSizes=modelDef.statesPerDelayedPose*modelDef.maxNumDelayedPoses,6*modelDef.maxNumDelayedPoses
  applyXstateErrors : Subsystem
  wires:
  errors/1 -> Selector1/1, Selector/1
  Selector/1 -> applyXstateErrors/1(errorStateEstimates)
  Selector1/1 -> Pad/1
  Data Store Read/1 -> For Each Subsystem/2(C_c_n_list_in)
  Data Store Read1/1 -> For Each Subsystem/3(r_c_n_list_in)
  For Each Subsystem/1(C_c_n_list) -> Data Store Write/1
  For Each Subsystem/2(r_c_n_list) -> Data Store Write1/1
  Pad/1 -> For Each Subsystem/1(delayedPoseCorrections)

== system VINS/measUpdate/relativePoseUpdate/get row indices/validateRecency ==
  In1 : Inport
  In2 : Inport  Port=2
  Assertion : Assertion
  Data Store Read : DataStoreRead  DataStoreName=newestDelayedPoseIdx
  Logical Operator : Logic  Operator=OR  AllPortsSameDT=off  OutDataTypeStr=boolean
  Logical Operator1 : Logic  Operator=OR  AllPortsSameDT=off  OutDataTypeStr=boolean
  Logical Operator2 : Logic  AllPortsSameDT=off  OutDataTypeStr=boolean
  Relational Operator{,1..3} (4 alike) : RelationalOperator  Operator===  OutDataTypeStr=boolean  RndMeth=Simplest
  Scope : Scope
  Scope1 : Scope
  previousIndex : Subsystem
  previousIndex1 : Subsystem
  valid : Outport
  wires:
  In1/1 -> Relational Operator3/2, Relational Operator1/1
  In2/1 -> Relational Operator2/1, Relational Operator/1
  previousIndex1/1(idx1) -> Relational Operator3/1
  Relational Operator3/1 -> Logical Operator1/2
  Relational Operator2/1 -> Logical Operator/2
  Logical Operator2/1 -> valid/1, Assertion/1
  Relational Operator1/1 -> Logical Operator1/1
  Relational Operator/1 -> Logical Operator/1
  previousIndex/1(idx1) -> previousIndex1/1(idx2), Relational Operator1/2, Relational Operator2/2
  Logical Operator1/1 -> Logical Operator2/2, Scope1/1
  Data Store Read/1 -> Relational Operator/2, previousIndex/1(idx2)  "idx2"
  Logical Operator/1 -> Logical Operator2/1, Scope/1

== system VINS/measUpdate/relativePoseUpdate/updateCovariance/repairCovarianceAndWrite ==
  In1 : Inport
  Data Store Write : DataStoreWrite  DataStoreName=Pxx
  Data Store Write1 : DataStoreWrite  DataStoreName=Pxc
  Data Store Write2 : DataStoreWrite  DataStoreName=Pcc
  LDL Factorization : dspfactors/LDL Factorization  errmode=Warning  roundingMode=Floor  overflowMode=off  outputMin=[]  outputMax=[]
      settings: SourceProductName=DSP System Toolbox  SourceProductBaseCode=DS
  Submatrix3 : dspmtrx3/Submatrix  RowSpan=Range of rows  RowStartMode=First  RowStartIndex=1  RowEndMode=Index  RowEndIndex=modelDef.numStates  ColSpan=Range of columns  ColStartMode=First  ColStartIndex=1  ColEndMode=Index  ColEndIndex=modelDef.numStates
  Submatrix4 : dspmtrx3/Submatrix  RowSpan=Range of rows  RowStartMode=First  RowStartIndex=1  RowEndMode=Index  RowEndIndex=modelDef.numStates  ColSpan=Range of columns  ColStartMode=Index  ColStartIndex=modelDef.numStates + 1  ColEndMode=Last  ColEndIndex=1
  Submatrix5 : dspmtrx3/Submatrix  RowSpan=Range of rows  RowStartMode=Index  RowStartIndex=modelDef.numStates + 1  RowEndMode=Last  RowEndIndex=modelDef.numStates  ColSpan=Range of columns  ColStartMode=Index  ColStartIndex=modelDef.numStates + 1  ColEndMode=Last  ColEndIndex=1
  lowerBoundDiagonal and reconstruct : Subsystem  TreatAsAtomicUnit=on
  wires:
  LDL Factorization/1 -> lowerBoundDiagonal and reconstruct/1(LDL')
  lowerBoundDiagonal and reconstruct/1(P) -> Submatrix5/1, Submatrix4/1, Submatrix3/1
  Submatrix3/1 -> Data Store Write/1
  Submatrix4/1 -> Data Store Write1/1
  Submatrix5/1 -> Data Store Write2/1
  In1/1 -> LDL Factorization/1

== system VINS/measUpdate/relativePoseUpdate/updateCovariance/writeCovariances ==
  In1 : Inport
  Data Store Write3 : DataStoreWrite  DataStoreName=Pxx
  Data Store Write4 : DataStoreWrite  DataStoreName=Pxc
  Data Store Write5 : DataStoreWrite  DataStoreName=Pcc
  Submatrix : dspmtrx3/Submatrix  RowSpan=Range of rows  RowStartMode=First  RowStartIndex=1  RowEndMode=Index  RowEndIndex=modelDef.numStates  ColSpan=Range of columns  ColStartMode=First  ColStartIndex=1  ColEndMode=Index  ColEndIndex=modelDef.numStates
  Submatrix1 : dspmtrx3/Submatrix  RowSpan=Range of rows  RowStartMode=First  RowStartIndex=1  RowEndMode=Index  RowEndIndex=modelDef.numStates  ColSpan=Range of columns  ColStartMode=Index  ColStartIndex=modelDef.numStates + 1  ColEndMode=Last  ColEndIndex=1
  Submatrix2 : dspmtrx3/Submatrix  RowSpan=Range of rows  RowStartMode=Index  RowStartIndex=modelDef.numStates + 1  RowEndMode=Last  RowEndIndex=modelDef.numStates  ColSpan=Range of columns  ColStartMode=Index  ColStartIndex=modelDef.numStates + 1  ColEndMode=Last  ColEndIndex=1
  lowerBoundStates : Subsystem  TreatAsAtomicUnit=on
  lowerBoundStates1 : Subsystem  TreatAsAtomicUnit=on
  wires:
  Submatrix/1 -> lowerBoundStates/1(In1)
  Submatrix2/1 -> lowerBoundStates1/1(In1)
  Submatrix1/1 -> Data Store Write4/1
  lowerBoundStates1/1(Out1) -> Data Store Write5/1
  lowerBoundStates/1(Out1) -> Data Store Write3/1
  In1/1 -> Submatrix2/1, Submatrix1/1, Submatrix/1

== system VINS/measUpdate/relocalize/Subsystem/norm ==
  In1 : Inport
  Math Function : Math  Operator=square  SaturateOnIntegerOverflow=on
  Math Function1 : Math  Operator=sqrt  SaturateOnIntegerOverflow=on
  Sum of Elements : Sum  Inputs=+
  Out1 : Outport
  wires:
  In1/1 -> Math Function/1
  Sum of Elements/1 -> Math Function1/1
  Math Function/1 -> Sum of Elements/1
  Math Function1/1 -> Out1/1

== system VINS/measUpdate/relocalize/Subsystem/setPosition ==
  r_nc_n : Inport
  yawChanged : Inport  Port=2
  Enable : EnablePort
  Constant10 : Constant  Value=0  OutDataTypeStr=Inherit: Inherit via back propagation
  Constant9 : Constant  Value=imuLocationMm  OutDataTypeStr=Inherit: Inherit via back propagation
  DT police3 : Subsystem  TreatAsAtomicUnit=on
  Data Store Read : DataStoreRead  DataStoreName=Cbn
  Data Store Write10 : DataStoreWrite  DataStoreName=distTravelled
  Data Store Write3 : DataStoreWrite  DataStoreName=rnav
  Gain : Gain  Gain=1/1000
  Matrix Multiply : Product  Multiplication=Matrix(*)
  Sum : Sum  Inputs=++|
  just to make sure yaw is updated first : Terminator
  wires:
  Sum/1 -> Data Store Write3/1  "r_nb_n"
  Matrix Multiply/1 -> Sum/1  "r_cb_n"
  Data Store Read/1 -> Matrix Multiply/1  "Ccn = Cbn"
  Constant9/1 -> Gain/1
  r_nc_n/1 -> Sum/2  "r_nc_n"
  Constant10/1 -> DT police3/1(In1), Data Store Write10/1
  Gain/1 -> Matrix Multiply/2  "r_cb_c"
  yawChanged/1 -> just to make sure yaw is updated first/1

== system VINS/measUpdate/relocalize/Subsystem/setYaw ==
  yaw : Inport
  Enable : EnablePort  ShowOutputPort=on
  Data Store Read : DataStoreRead  DataStoreName=Cbn
  Data Store Write3 : DataStoreWrite  DataStoreName=Cbn
  Demux : Demux  Outputs=3
  MATLAB Function3 : MATLAB Function  TreatAsAtomicUnit=on
  Mux : Mux  Inputs=3
  Permute Dimensions : PermuteDimensions
  Terminator : Terminator
  euler2dcm : MATLAB Function  TreatAsAtomicUnit=on
  yawChanged : Outport
  wires:
  Data Store Read/1 -> MATLAB Function3/1(Cbn)  "Ccn = Cbn"
  MATLAB Function3/1(eul) -> Demux/1
  Demux/1 -> Mux/1
  Demux/2 -> Mux/2
  yaw/1 -> Mux/3
  Demux/3 -> Terminator/1
  Mux/1 -> euler2dcm/1(eul_vect)
  euler2dcm/1(DCMnb) -> Permute Dimensions/1
  Permute Dimensions/1 -> Data Store Write3/1
  Enable/1 -> yawChanged/1

== system VINS/measUpdate/wipe out delayed states/setP/DT police1 ==
  In1 : Inport
  Data Store Read : DataStoreRead  DataStoreName=DataTypeRef
  Data Type Duplicate : DataTypeDuplicate
  wires:
  Data Store Read/1 -> Data Type Duplicate/1
  In1/1 -> Data Type Duplicate/2

== system VINS/measUpdate/wipe out delayed states/setP/DT police2 ==
  In1 : Inport
  Data Store Read : DataStoreRead  DataStoreName=DataTypeRef
  Data Type Duplicate : DataTypeDuplicate
  wires:
  In1/1 -> Data Type Duplicate/2
  Data Store Read/1 -> Data Type Duplicate/1

== system VINS/measUpdate/wipe out delayed states/setP/DT police3 ==
  In1 : Inport
  Data Store Read : DataStoreRead  DataStoreName=DataTypeRef
  Data Type Duplicate : DataTypeDuplicate
  wires:
  Data Store Read/1 -> Data Type Duplicate/1
  In1/1 -> Data Type Duplicate/2

== system VINS/measUpdate/zuptMeasUpdate/applyErrors/reOrthonormalization ==
  note: from http://www.dtic.mil/dtic/tr/fulltext/u2/p003621.pdf page 12
  note: Cfixed = C + 0.5(I-CC')C
  In1 : Inport
  C*C' : Product  Multiplication=Matrix(*)
  C*C'1 : Product  Multiplication=Matrix(*)
  Constant : Constant  Value=eye(3)  OutDataTypeStr=Inherit: Inherit via back propagation
  Gain : Gain  Gain=1/2
  Permute Dimensions : PermuteDimensions
  Sum : Sum  Inputs=|++
  Sum1 : Sum  Inputs=|+-
  Out1 : Outport
  wires:
  In1/1 -> Permute Dimensions/1, C*C'/1, C*C'1/2, Sum/1
  Sum/1 -> Out1/1
  Permute Dimensions/1 -> C*C'/2
  C*C'/1 -> Sum1/2
  Constant/1 -> Sum1/1
  Gain/1 -> Sum/2
  Sum1/1 -> C*C'1/1
  C*C'1/1 -> Gain/1

== system VINS/measUpdate/zuptMeasUpdate/applyErrors/updateAccelBiases ==
  In1 : Inport
  Enable : EnablePort
  Data Store Read5 : DataStoreRead  DataStoreName=df
  Data Store Write5 : DataStoreWrite  DataStoreName=df
  Sum4 : Sum  Inputs=++|
  wires:
  In1/1 -> Sum4/1
  Data Store Read5/1 -> Sum4/2
  Sum4/1 -> Data Store Write5/1

== system VINS/measUpdate/zuptMeasUpdate/applyErrors/updateAccelSfma ==
  In1 : Inport
  Enable : EnablePort
  " LU Inverse" : dspinverses/ LU Inverse
      settings: SourceProductName=DSP System Toolbox
  Bias : Bias  Bias=eye(3)
  Data Store Read6 : DataStoreRead  DataStoreName=Macc
  Data Store Write6 : DataStoreWrite  DataStoreName=Macc
  Data Store Write9 : DataStoreWrite  DataStoreName=IplusMinv_acc
  Reshape : Reshape  OutputDimensionality=Customize  OutputDimensions=[3,3]
  Sum5 : Sum  Inputs=++|
  wires:
  " LU Inverse"/1 -> Data Store Write9/1
  Bias/1 -> " LU Inverse"/1
  In1/1 -> Reshape/1
  Reshape/1 -> Sum5/1
  Data Store Read6/1 -> Sum5/2
  Sum5/1 -> Data Store Write6/1, Bias/1

== system VINS/measUpdate/zuptMeasUpdate/applyErrors/updateGyroGsensitivity ==
  In1 : Inport
  Enable : EnablePort
  Data Store Read7 : DataStoreRead  DataStoreName=Ggyr
  Data Store Write7 : DataStoreWrite  DataStoreName=Ggyr
  Reshape1 : Reshape  OutputDimensionality=Customize  OutputDimensions=[3,3]
  Sum6 : Sum  Inputs=++|
  wires:
  Data Store Read7/1 -> Sum6/2
  Reshape1/1 -> Sum6/1
  In1/1 -> Reshape1/1
  Sum6/1 -> Data Store Write7/1

== system VINS/measUpdate/zuptMeasUpdate/applyErrors/updateGyroSfma ==
  In1 : Inport
  Enable : EnablePort
  " LU Inverse1" : dspinverses/ LU Inverse
      settings: SourceProductName=DSP System Toolbox
  Bias1 : Bias  Bias=eye(3)
  Data Store Read7 : DataStoreRead  DataStoreName=Mgyr
  Data Store Write7 : DataStoreWrite  DataStoreName=Mgyr
  Data Store Write8 : DataStoreWrite  DataStoreName=IplusMinv_gyr
  Reshape1 : Reshape  OutputDimensionality=Customize  OutputDimensions=[3,3]
  Sum6 : Sum  Inputs=++|
  wires:
  " LU Inverse1"/1 -> Data Store Write8/1
  Bias1/1 -> " LU Inverse1"/1
  Data Store Read7/1 -> Sum6/2
  Reshape1/1 -> Sum6/1
  In1/1 -> Reshape1/1
  Sum6/1 -> Data Store Write7/1, Bias1/1

== system VINS/measUpdate/absolutePoseUpdate/applyErrors/For Each Subsystem/reOrthonormalization ==
  note: from http://www.dtic.mil/dtic/tr/fulltext/u2/p003621.pdf page 12
  note: Cfixed = C + 0.5(I-CC')C
  In1 : Inport
  C*C' : Product  Multiplication=Matrix(*)
  C*C'1 : Product  Multiplication=Matrix(*)
  Constant : Constant  Value=eye(3)  OutDataTypeStr=Inherit: Inherit via back propagation
  Gain : Gain  Gain=1/2
  Permute Dimensions : PermuteDimensions
  Sum : Sum  Inputs=|++
  Sum1 : Sum  Inputs=|+-
  Out1 : Outport
  wires:
  In1/1 -> Permute Dimensions/1, C*C'/1, C*C'1/2, Sum/1
  Sum/1 -> Out1/1
  Permute Dimensions/1 -> C*C'/2
  C*C'/1 -> Sum1/2
  Constant/1 -> Sum1/1
  Gain/1 -> Sum/2
  Sum1/1 -> C*C'1/1
  C*C'1/1 -> Gain/1
